simulink model "neha_project"  (Simulink 7.3)
settings: Solver=ode23tb  StartTime=0.0  StopTime=5  RelTol=1000e-2
undefined symbols (not defined in the file): DiscIntNeverNeededParam
libraries: powerlib x16
settings Model: Creator=jassi  LastModifiedBy=ankit
settings SolverCC: ShapePreserveControl=EnableAll  ZeroCrossControl=DisableAll

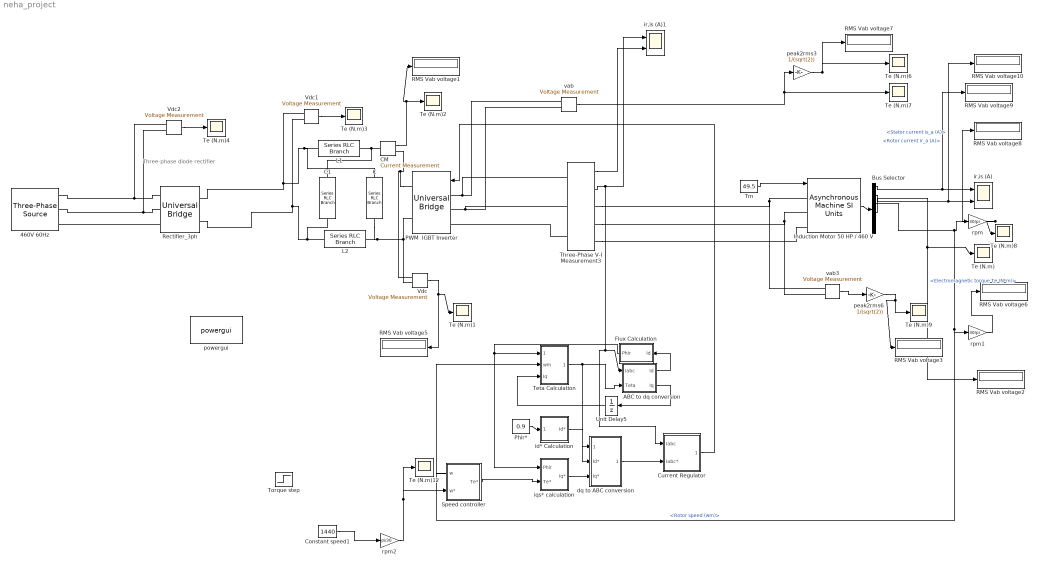
== system neha_project ==
  note: Three-phase
      | diode rectifier
  460V 60Hz : powerlib/Electrical Sources/Three-Phase Source  DialogController=POWERSYS.PowerSysDialog  SystemSampleTime=-1  Voltage=460  PhaseAngle=0  Frequency=50  InternalConnection=Yg  SpecifyImpedance=off  Resistance=0.1  Inductance=1.2e-3  ShortCircuitLevel=100e6  BaseVoltage=25e3  XRratio=7
  ABC to dq conversion : Subsystem
  Bus Selector : BusSelector  OutputSignals=Rotor measurements.Rotor current ir_a (A),Stator measurements.Stator current is_a (A),Mechanical.Rotor speed (wm),Mechanical.Electromagnetic torque Te (N*m),Stator measurements.Stator flux phis_q (V s),Stator measurements.Stator flux phis_d (V s)
  "C " : powerlib/Elements/Series RLC Branch  DialogController=POWERSYS.PowerSysDialog  PhysicalDomain=powersysdomain  SubClassName=unknown  LeftPortType=p1  RightPortType=p1  LConnTagsString=__new0  RConnTagsString=__new0  BranchType=C  Resistance=1  Inductance=1e-3  SetiL0=off  InitialCurrent=0  Capacitance=0.05  Setx0=off  InitialVoltage=0  Measurements=None
  "C1 " : powerlib/Elements/Series RLC Branch  DialogController=POWERSYS.PowerSysDialog  PhysicalDomain=powersysdomain  SubClassName=unknown  LeftPortType=p1  RightPortType=p1  LConnTagsString=__new0  RConnTagsString=__new0  BranchType=C  Resistance=1  Inductance=1e-3  SetiL0=off  InitialCurrent=0  Capacitance=0.05  Setx0=off  InitialVoltage=0  Measurements=None
  CM : powerlib/Measurements/Current Measurement  DialogController=POWERSYS.PowerSysDialog  SystemSampleTime=-1  PhasorSimulation=off  OutputType=Complex  PSBequivalent=0
  Constant speed1 : Constant  Value=1440  OutDataType=sfix(16)  OutScaling=2^0
  Current Regulator : Subsystem  mask(Regulateur de courant a hysteresis){h=20}
      mask prompts: h "Hysteresis band (A)"
  Flux Calculation : Subsystem  mask(Flux Calcultation){}
      mask init:
      | NF=0.44572610323020e-6;
      | DF=[1 -0.99998715486734];
  Induction Motor 50 HP / 460 V : powerlib/Machines/Asynchronous Machine SI Units  DialogController=POWERSYS.PowerSysDialog  SystemSampleTime=-1  PresetModel=No  MechanicalLoad=Torque Tm  ShowDetailedParameters=on  RotorType=Squirrel-cage  ReferenceFrame=Stationary  NominalParameters=[ 7.5e3, 460,50]  Stator=[ 0.6 4.5e-3 ]  Rotor=[ 0.7 4.5e-3 ]  Lm=80e-3  Mechanical=[0.1 0.01 2 ]  PolePairs=2  InitialConditions="[ 1, 0 ,  0 , 0 , 0 , 0 , 0 , 0 ]"  Units=SI  LoadFlowParameters=0  SimulateSaturation=off  Saturation=[0 0;0 0]  TsPowergui=0  TsBlock=-1  IterativeModel=Trapezoidal non iterative
  L1 : powerlib/Elements/Series RLC Branch  DialogController=POWERSYS.PowerSysDialog  PhysicalDomain=powersysdomain  SubClassName=unknown  LeftPortType=p1  RightPortType=p1  LConnTagsString=__new0  RConnTagsString=__new0  BranchType=L  Resistance=1  Inductance=4e-9  SetiL0=off  InitialCurrent=0  Capacitance=1e-6  Setx0=off  InitialVoltage=0  Measurements=None
  L2 : powerlib/Elements/Series RLC Branch  DialogController=POWERSYS.PowerSysDialog  PhysicalDomain=powersysdomain  SubClassName=unknown  LeftPortType=p1  RightPortType=p1  LConnTagsString=__new0  RConnTagsString=__new0  BranchType=L  Resistance=1  Inductance=4e-9  SetiL0=off  InitialCurrent=0  Capacitance=1e-6  Setx0=off  InitialVoltage=0  Measurements=None
  PWM  IGBT Inverter : powerlib/Power Electronics/Universal Bridge  DialogController=POWERSYS.PowerSysDialog  SystemSampleTime=-1  Arms=3  SnubberResistance=1000  SnubberCapacitance=inf  Device=IGBT / Diodes  Ron=1e-3  Lon=0  ForwardVoltages="[  0.0  0.0  ]"  ForwardVoltage=.8  GTOparameters=[ 1e-6 ,1e-6 ]  IGBTparameters=[ 1e-6 , 2.144e-6 ]  Measurements=None  Measurements_2=None  converterType=Rectifier
  Phir* : Constant  Value=0.9  OutDataType=sfix(16)  OutScaling=2^0
  RMS Vab voltage{1..3,5..10} (9 alike) : Display
      settings: Decimation=100
  Rectifier_3ph : powerlib/Power Electronics/Universal Bridge  DialogController=POWERSYS.PowerSysDialog  SystemSampleTime=-1  Arms=3  SnubberResistance=10e3  SnubberCapacitance=20e-9  Device=Diodes  Ron=1e-3  Lon=0  ForwardVoltages="[  0,  0  ]"  ForwardVoltage=1.3  GTOparameters=[ 10e-6, 20e-6 ]  IGBTparameters=[ 1e-6 , 2e-6 ]  Measurements=All voltages and currents  Measurements_2=None  converterType=Rectifier
  Speed controller : Subsystem  mask(PI controller){Kp=4, Ki=200, Tlim=200, Ts=2e-006}
      mask prompts: Kp "Proportional gain (Kp)"; Ki "Integral gain (Ki)"; Tlim "Torque limit (N.m)"; Ts "Sampling time (s)"
      mask help: Proportional-Integral Speed Controller
      mask Display: plot(0,0,100,100,[35,35,65],[70,30,30],[35,65],[45,60])
  Te (N.m){,1..4,6..9,12} (10 alike) : Scope
      Te (N.m) settings: YMin=20  YMax=75  SaveName=ScopeData2  DataFormat=Structure
      Te (N.m)1 settings: YMin=510  YMax=690  SaveName=ScopeData8  DataFormat=Structure
      Te (N.m)12 settings: YMin=120  YMax=120  SaveName=ScopeData16  DataFormat=Structure
      Te (N.m)2 settings: YMin=-40  YMax=60  SaveName=ScopeData9  DataFormat=Structure
      Te (N.m)3 settings: YMin=588  YMax=603  SaveName=ScopeData10  DataFormat=Structure
      Te (N.m)4 settings: YMin=-450  YMax=450  SaveName=ScopeData3  DataFormat=Structure
      Te (N.m)6 settings: YMin=-450  YMax=25  SaveName=ScopeData12  DataFormat=Structure
      Te (N.m)7 settings: YMin=-700  YMax=700  SaveName=ScopeData13  DataFormat=Structure
      Te (N.m)8 settings: TimeRange=1  YMin=550  YMax=1600  DataFormat=Structure
      Te (N.m)9 settings: TimeRange=1  YMin=-400  YMax=400  SaveName=ScopeData14  DataFormat=Structure
  Teta Calculation : Subsystem
  Three-Phase V-I Measurement3 : powerlib/Measurements/Three-Phase V-I Measurement  DialogController=POWERSYS.PowerSysDialog  SystemSampleTime=-1  VoltageMeasurement=phase-to-phase  SetLabelV=off  LabelV=Vabc  Vpu=off  CurrentMeasurement=yes  SetLabelI=off  LabelI=Iabc  Ipu=off  Pbase=100e6  Vbase=500e3  OutputType=Complex  PhasorSimulation=off  PSBequivalent=0
  Tm : Constant  Value=49.5  OutDataType=sfix(16)  OutScaling=2^0
  Torque step : Step  Time=1.8  After=200  SampleTime=0
  Unit Delay5 : UnitDelay  SampleTime=2e-006
  Vdc : powerlib/Measurements/Voltage Measurement  Tag=PoWeRsYsTeMmEaSuReMeNt  DialogController=POWERSYS.PowerSysDialog  SystemSampleTime=-1  PhasorSimulation=off  OutputType=Magnitude  PSBequivalent=0
  Vdc1 : powerlib/Measurements/Voltage Measurement  Tag=PoWeRsYsTeMmEaSuReMeNt  DialogController=POWERSYS.PowerSysDialog  SystemSampleTime=-1  PhasorSimulation=off  OutputType=Magnitude  PSBequivalent=0
  Vdc2 : powerlib/Measurements/Voltage Measurement  Tag=PoWeRsYsTeMmEaSuReMeNt  DialogController=POWERSYS.PowerSysDialog  SystemSampleTime=-1  PhasorSimulation=off  OutputType=Magnitude  PSBequivalent=0
  dq to ABC conversion : Subsystem
  id* Calculation : Subsystem
  iqs* calculation : Subsystem
  ir,is (A) : Scope  NumInputPorts=2
      settings: YMin=-27.5~-55  YMax=17.5~50  DataFormat=Structure
  ir,is (A)1 : Scope  NumInputPorts=2
      settings: YMin=-27.5~-700  YMax=27.5~700  SaveName=ScopeData17  DataFormat=Structure
  peak2rms3 : Gain  Gain=1/(sqrt(2))  ParameterDataType=sfix(16)  ParameterScaling=2^0  OutDataType=sfix(16)  OutScaling=2^0  SaturateOnIntegerOverflow=on  OutDataTypeStr=Inherit: Same as input  ParamDataTypeStr=Inherit: Same as input
  peak2rms6 : Gain  Gain=1/(sqrt(2))  ParameterDataType=sfix(16)  ParameterScaling=2^0  OutDataType=sfix(16)  OutScaling=2^0  SaturateOnIntegerOverflow=on  OutDataTypeStr=Inherit: Same as input  ParamDataTypeStr=Inherit: Same as input
  powergui : powerlib/powergui  Priority=2  SystemSampleTime=-1  SimulationMode=Discrete  SampleTime=2e-006  frequency=60  SPID=off  DisableSnubberDevices=off  DisableRonSwitches=off  DisableVfSwitches=off  SwTol=0  Interpol=off  frequencyindice=50  echomessages=off  HookPort=off  DisplayEquations=off  FunctionMessages=off  EnableUseOfTLC=off  x0status=blocks  RestoreLinks=warning  Frange=[0:2:500]  Ylog=off  Xlog=on  ShowGrid=off  save=off  variable=ZData  ZoomFFT=on  StartTime=0.0  cycles=1  DisplayStyle=off  fundamental=60  FreqAxis=off  MaxFrequency=1000  frequencyindicesteady=1  RmsSteady=1  display=off  Ts=0  methode=off
  rpm : Gain  Gain=30/pi  ParameterDataType=sfix(16)  ParameterScaling=2^0  OutDataType=sfix(16)  OutScaling=2^0  SaturateOnIntegerOverflow=on  OutDataTypeStr=Inherit: Same as input  ParamDataTypeStr=Inherit: Same as input
  rpm1 : Gain  Gain=30/pi  ParameterDataType=sfix(16)  ParameterScaling=2^0  OutDataType=sfix(16)  OutScaling=2^0  SaturateOnIntegerOverflow=on  OutDataTypeStr=Inherit: Same as input  ParamDataTypeStr=Inherit: Same as input
  rpm2 : Gain  Gain=pi/30  ParameterDataType=sfix(16)  ParameterScaling=2^0  OutDataType=sfix(16)  OutScaling=2^0  SaturateOnIntegerOverflow=on  OutDataTypeStr=Inherit: Same as input  ParamDataTypeStr=Inherit: Same as input
  vab : powerlib/Measurements/Voltage Measurement  Tag=PoWeRsYsTeMmEaSuReMeNt  DialogController=POWERSYS.PowerSysDialog  SystemSampleTime=-1  PhasorSimulation=off  OutputType=Magnitude  PSBequivalent=0
  vab3 : powerlib/Measurements/Voltage Measurement  Tag=PoWeRsYsTeMmEaSuReMeNt  DialogController=POWERSYS.PowerSysDialog  SystemSampleTime=-1  PhasorSimulation=off  OutputType=Magnitude  PSBequivalent=0
  wires:
  Bus Selector/4 -> Te (N.m)/1, RMS Vab voltage2/1  "<Electromagnetic torque Te (N*m)>"
  Bus Selector/1 -> RMS Vab voltage9/1, ir,is (A)/1  "<Rotor current ir_a (A)>"
  Induction Motor 50 HP / 460 V/1 -> Bus Selector/1
  Bus Selector/2 -> ir,is (A)/2, RMS Vab voltage10/1  "<Stator current is_a (A)>"
  vab/1 -> peak2rms3/1, Te (N.m)7/1
  Tm/1 -> Induction Motor 50 HP / 460 V/1
  peak2rms3/1 -> Te (N.m)6/1, RMS Vab voltage7/1
  peak2rms6/1 -> RMS Vab voltage3/1, Te (N.m)9/1
  Vdc/1 -> Te (N.m)1/1, RMS Vab voltage5/1
  CM/1 -> Te (N.m)2/1, RMS Vab voltage1/1
  Vdc1/1 -> Te (N.m)3/1
  Three-Phase V-I Measurement3/1 -> ir,is (A)1/2
  Three-Phase V-I Measurement3/2 -> ir,is (A)1/1, Current Regulator/1(Iabc), ABC to dq conversion/1(Iabc)
  vab3/1 -> peak2rms6/1
  Current Regulator/1(Pulses) -> PWM  IGBT Inverter/1
  Bus Selector/3 -> rpm/1, rpm1/1, Teta Calculation/2(wm), Speed controller/1(w)  "<Rotor speed (wm)>"
  rpm/1 -> RMS Vab voltage8/1, Te (N.m)8/1
  rpm1/1 -> RMS Vab voltage6/1
  Teta Calculation/1(Teta) -> dq to ABC conversion/1(Teta), ABC to dq conversion/2(Teta)
  iqs* calculation/1(Iq*) -> dq to ABC conversion/3(Iq*)
  Unit Delay5/1 -> Teta Calculation/3(Iq)
  ABC to dq conversion/2(Iq) -> Unit Delay5/1
  Flux Calculation/1(Phir) -> Teta Calculation/1(Phir), iqs* calculation/1(Phir)
  id* Calculation/1(Id*) -> dq to ABC conversion/2(Id*)
  ABC to dq conversion/1(Id) -> Flux Calculation/1(Id)
  Phir*/1 -> id* Calculation/1(Phir*)
  Speed controller/1(Te*) -> iqs* calculation/2(Te*)
  dq to ABC conversion/1(Iabc*) -> Current Regulator/2(Iabc*)
  rpm2/1 -> Te (N.m)12/1, Speed controller/2(w*)
  Constant speed1/1 -> rpm2/1
  Vdc2/1 -> Te (N.m)4/1
  connections:
  L1/RConn1 -- CM/LConn1 -- "C1 "/LConn1
  Rectifier_3ph/RConn1 -- Vdc1/LConn1 -- L1/LConn1 -- "C "/LConn1
  PWM  IGBT Inverter/RConn2 -- Vdc/LConn2 -- "C "/RConn1 -- L2/RConn1
  Rectifier_3ph/RConn2 -- Vdc1/LConn2 -- L2/LConn1 -- "C1 "/RConn1
  PWM  IGBT Inverter/RConn1 -- Vdc/LConn1 -- CM/RConn1
  Three-Phase V-I Measurement3/RConn2 -- Induction Motor 50 HP / 460 V/LConn2 -- vab3/LConn2
  Three-Phase V-I Measurement3/RConn3 -- Induction Motor 50 HP / 460 V/LConn3
  Three-Phase V-I Measurement3/LConn1 -- PWM  IGBT Inverter/LConn1 -- vab/LConn1
  Three-Phase V-I Measurement3/LConn2 -- vab/LConn2 -- PWM  IGBT Inverter/LConn2
  Three-Phase V-I Measurement3/LConn3 -- PWM  IGBT Inverter/LConn3
  Three-Phase V-I Measurement3/RConn1 -- Induction Motor 50 HP / 460 V/LConn1 -- vab3/LConn1
  460V 60Hz/RConn1 -- Rectifier_3ph/LConn1 -- Vdc2/LConn1
  Rectifier_3ph/LConn3 -- 460V 60Hz/RConn3
  460V 60Hz/RConn2 -- Rectifier_3ph/LConn2 -- Vdc2/LConn2

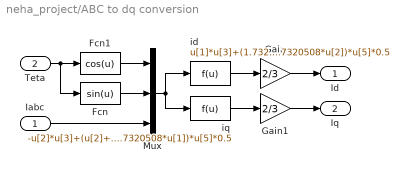
== system neha_project/ABC to dq conversion ==
  Iabc : Inport  OutDataType=sfix(16)  OutScaling=2^0
  Teta : Inport  Port=2  OutDataType=sfix(16)  OutScaling=2^0
  Fcn : Fcn  Expr=sin(u)
  Fcn1 : Fcn  Expr=cos(u)
  Gain : Gain  Gain=2/3  ParameterDataType=sfix(16)  ParameterScaling=2^0  OutDataType=sfix(16)  OutScaling=2^0  SaturateOnIntegerOverflow=on  OutDataTypeStr=Inherit: Same as input  ParamDataTypeStr=Inherit: Same as input
  Gain1 : Gain  Gain=2/3  ParameterDataType=sfix(16)  ParameterScaling=2^0  OutDataType=sfix(16)  OutScaling=2^0  SaturateOnIntegerOverflow=on  OutDataTypeStr=Inherit: Same as input  ParamDataTypeStr=Inherit: Same as input
  Mux : Mux  Inputs=[1 1 3]
  id : Fcn  Expr=u[1]*u[3]+(1.7320508*u[2]-u[1])*u[4]*0.5+(-u[1]-1.7320508*u[2])*u[5]*0.5
  iq : Fcn  Expr=-u[2]*u[3]+(u[2]+1.7320508*u[1])*u[4]*0.5+(u[2]-1.7320508*u[1])*u[5]*0.5
  Id : Outport  OutDataType=sfix(16)  OutScaling=2^0  InitialOutput=0
  Iq : Outport  Port=2  OutDataType=sfix(16)  OutScaling=2^0  InitialOutput=0
  wires:
  Fcn/1 -> Mux/2
  Fcn1/1 -> Mux/1
  Teta/1 -> Fcn1/1, Fcn/1
  Mux/1 -> iq/1, id/1
  Iabc/1 -> Mux/3
  iq/1 -> Gain1/1
  id/1 -> Gain/1
  Gain/1 -> Id/1
  Gain1/1 -> Iq/1

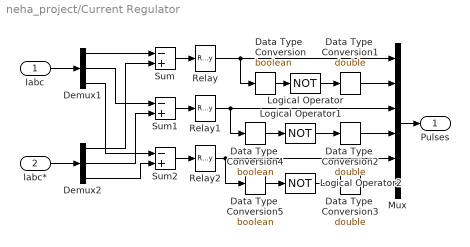
== system neha_project/Current Regulator ==
  Iabc : Inport  OutDataType=sfix(16)  OutScaling=2^0
  Iabc* : Inport  Port=2  OutDataType=sfix(16)  OutScaling=2^0
  Data Type  Conversion : DataTypeConversion  OutDataTypeMode=boolean  OutDataType=sfix(16)  OutScaling=2^0  OutDataTypeStr=boolean  SaturateOnIntegerOverflow=on  RndMeth=Zero
  Data Type  Conversion1 : DataTypeConversion  OutDataTypeMode=double  OutDataType=sfix(16)  OutScaling=2^0  OutDataTypeStr=double  SaturateOnIntegerOverflow=on  RndMeth=Zero
  Data Type  Conversion2 : DataTypeConversion  OutDataTypeMode=double  OutDataType=sfix(16)  OutScaling=2^0  OutDataTypeStr=double  SaturateOnIntegerOverflow=on  RndMeth=Zero
  Data Type  Conversion3 : DataTypeConversion  OutDataTypeMode=double  OutDataType=sfix(16)  OutScaling=2^0  OutDataTypeStr=double  SaturateOnIntegerOverflow=on  RndMeth=Zero
  Data Type  Conversion4 : DataTypeConversion  OutDataTypeMode=boolean  OutDataType=sfix(16)  OutScaling=2^0  OutDataTypeStr=boolean  SaturateOnIntegerOverflow=on  RndMeth=Zero
  Data Type  Conversion5 : DataTypeConversion  OutDataTypeMode=boolean  OutDataType=sfix(16)  OutScaling=2^0  OutDataTypeStr=boolean  SaturateOnIntegerOverflow=on  RndMeth=Zero
  Demux1 : Demux  Outputs=3
  Demux2 : Demux  Outputs=3
  Logical Operator : Logic  Operator=NOT
  Logical Operator1 : Logic  Operator=NOT
  Logical Operator2 : Logic  Operator=NOT
  Mux : Mux  Inputs=6
  Relay : Relay  OnSwitchValue=h/2  OffSwitchValue=-h/2  OutDataType=sfix(16)  OutScaling=2^0
  Relay1 : Relay  OnSwitchValue=h/2  OffSwitchValue=-h/2  OutDataType=sfix(16)  OutScaling=2^0
  Relay2 : Relay  OnSwitchValue=h/2  OffSwitchValue=-h/2  OutDataType=sfix(16)  OutScaling=2^0
  Sum : Sum  Inputs=-+  OutDataType=sfix(16)  OutScaling=2^0  SaturateOnIntegerOverflow=on  InputSameDT=on  OutDataTypeStr=Inherit: Same as first input
  Sum1 : Sum  Inputs=-+  OutDataType=sfix(16)  OutScaling=2^0  SaturateOnIntegerOverflow=on  InputSameDT=on  OutDataTypeStr=Inherit: Same as first input
  Sum2 : Sum  Inputs=-+  OutDataType=sfix(16)  OutScaling=2^0  SaturateOnIntegerOverflow=on  InputSameDT=on  OutDataTypeStr=Inherit: Same as first input
  Pulses : Outport  OutDataType=sfix(16)  OutScaling=2^0  InitialOutput=0
  wires:
  Sum/1 -> Relay/1
  Sum1/1 -> Relay1/1
  Demux1/1 -> Sum/1
  Demux1/2 -> Sum1/1
  Mux/1 -> Pulses/1
  Iabc/1 -> Demux1/1
  Sum2/1 -> Relay2/1
  Demux1/3 -> Sum2/1
  Demux2/3 -> Sum2/2
  Demux2/2 -> Sum1/2
  Demux2/1 -> Sum/2
  Iabc*/1 -> Demux2/1
  Relay/1 -> Mux/1, Data Type  Conversion/1
  Relay1/1 -> Mux/3, Data Type  Conversion4/1
  Relay2/1 -> Mux/5, Data Type  Conversion5/1
  Data Type  Conversion/1 -> Logical Operator/1
  Logical Operator/1 -> Data Type  Conversion1/1
  Data Type  Conversion1/1 -> Mux/2
  Logical Operator1/1 -> Data Type  Conversion2/1
  Data Type  Conversion2/1 -> Mux/4
  Logical Operator2/1 -> Data Type  Conversion3/1
  Data Type  Conversion3/1 -> Mux/6
  Data Type  Conversion4/1 -> Logical Operator1/1
  Data Type  Conversion5/1 -> Logical Operator2/1

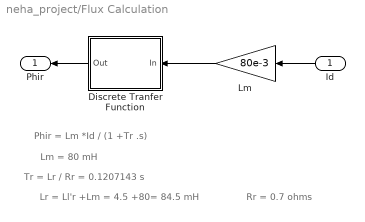
== system neha_project/Flux Calculation ==
  note: Phir = Lm *Id / (1 +Tr .s)
  note: Lm = 80 mH
  note: Lr = Ll'r +Lm = 4.5 +80= 84.5 mH
  note: Tr = Lr / Rr = 0.1207143 s
  note: Rr = 0.7 ohms
  Id : Inport  OutDataType=sfix(16)  OutScaling=2^0
  Discrete Tranfer Function : Subsystem  mask(First Order Low Pass Filter (Discrete)){T=0.1207143, Ts=2e-006}
      mask prompts: T "Time constant T (s) :"; Ts "Time step (s)"
      mask help: H(s)=1/(1+T.s)
      mask init:
      | X=[0 1 2 3 4];
      |  Y=[-2 -2 -3 -4 -4];
      |  str=sprintf('\nH=1/(1+T.s)\n T= %g s\n\n\n',T);
      | num=1;
      | den=[T 1];
      | 
      | % discrete transfer function
      | % descending powers of z
      | numd= Ts/T;
      | dend=[ 1  (Ts-T)/T];
      mask Display:
      | plot(X,Y);
      | disp(str);
  Lm : Gain  Gain=80e-3  ParameterDataType=sfix(16)  ParameterScaling=2^0  OutDataType=sfix(16)  OutScaling=2^0  SaturateOnIntegerOverflow=on  OutDataTypeStr=Inherit: Same as input  ParamDataTypeStr=Inherit: Same as input
  Phir : Outport  OutDataType=sfix(16)  OutScaling=2^0
  wires:
  Discrete Tranfer Function/1(Out) -> Phir/1
  Id/1 -> Lm/1
  Lm/1 -> Discrete Tranfer Function/1(In)

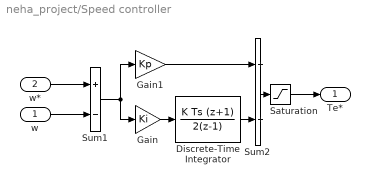
== system neha_project/Speed controller ==
  w : Inport  OutDataType=sfix(16)  OutScaling=2^0
  w* : Inport  Port=2  OutDataType=sfix(16)  OutScaling=2^0
  Discrete-Time Integrator : DiscreteIntegrator  IntegratorMethod=Integration: Trapezoidal  SampleTime=Ts  OutDataType=sfix(16)  OutScaling=2^0  LimitOutput=on  UpperSaturationLimit=Tlim  LowerSaturationLimit=-Tlim  ICPrevOutput=DiscIntNeverNeededParam  ICPrevScaledInput=DiscIntNeverNeededParam
  Gain : Gain  Gain=Ki  ParameterDataType=sfix(16)  ParameterScaling=2^0  OutDataType=sfix(16)  OutScaling=2^0  SaturateOnIntegerOverflow=on  OutDataTypeStr=Inherit: Same as input  ParamDataTypeStr=Inherit: Same as input
  Gain1 : Gain  Gain=Kp  ParameterDataType=sfix(16)  ParameterScaling=2^0  OutDataType=sfix(16)  OutScaling=2^0  SaturateOnIntegerOverflow=on  OutDataTypeStr=Inherit: Same as input  ParamDataTypeStr=Inherit: Same as input
  Saturation : Saturate  UpperLimit=Tlim  LowerLimit=-Tlim
  Sum1 : Sum  Inputs=+-  OutDataType=sfix(16)  OutScaling=2^0  SaturateOnIntegerOverflow=on  InputSameDT=on  OutDataTypeStr=Inherit: Same as first input
  Sum2 : Sum  OutDataType=sfix(16)  OutScaling=2^0  SaturateOnIntegerOverflow=on  InputSameDT=on  OutDataTypeStr=Inherit: Same as first input
  Te* : Outport  OutDataType=sfix(16)  OutScaling=2^0  InitialOutput=0
  wires:
  Gain1/1 -> Sum2/1
  Gain/1 -> Discrete-Time Integrator/1
  Sum1/1 -> Gain/1, Gain1/1
  Discrete-Time Integrator/1 -> Sum2/2
  Sum2/1 -> Saturation/1
  Saturation/1 -> Te*/1
  w/1 -> Sum1/2
  w*/1 -> Sum1/1

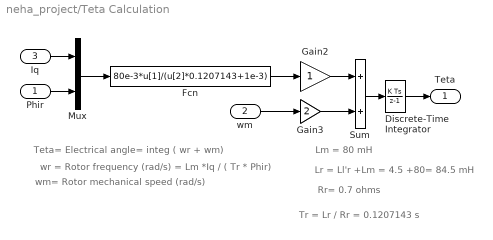
== system neha_project/Teta Calculation ==
  note: Teta= Electrical angle= integ ( wr + wm)
  note: wr = Rotor frequency (rad/s) = Lm *Iq / ( Tr * Phir)
  note: Lm = 80 mH
  note: Rr= 0.7 ohms
  note: Lr = Ll'r +Lm = 4.5 +80= 84.5 mH
  note: wm= Rotor mechanical speed (rad/s)
  note: Tr = Lr / Rr = 0.1207143 s
  Phir : Inport  OutDataType=sfix(16)  OutScaling=2^0
  wm : Inport  Port=2  OutDataType=sfix(16)  OutScaling=2^0
  Iq : Inport  Port=3  OutDataType=sfix(16)  OutScaling=2^0
  Discrete-Time Integrator : DiscreteIntegrator  SampleTime=2e-6  OutDataType=sfix(16)  OutScaling=2^0  ICPrevOutput=DiscIntNeverNeededParam  ICPrevScaledInput=DiscIntNeverNeededParam
  Fcn : Fcn  Expr=80e-3*u[1]/(u[2]*0.1207143+1e-3)
  Gain2 : Gain  ParameterDataType=sfix(16)  ParameterScaling=2^0  OutDataType=sfix(16)  OutScaling=2^0  SaturateOnIntegerOverflow=on  OutDataTypeStr=Inherit: Same as input  ParamDataTypeStr=Inherit: Same as input
  Gain3 : Gain  Gain=2  ParameterDataType=sfix(16)  ParameterScaling=2^0  OutDataType=sfix(16)  OutScaling=2^0  SaturateOnIntegerOverflow=on  OutDataTypeStr=Inherit: Same as input  ParamDataTypeStr=Inherit: Same as input
  Mux : Mux  Inputs=2
  Sum : Sum  OutDataType=sfix(16)  OutScaling=2^0  SaturateOnIntegerOverflow=on  InputSameDT=on  OutDataTypeStr=Inherit: Same as first input
  Teta : Outport  OutDataType=sfix(16)  OutScaling=2^0  InitialOutput=0
  wires:
  Discrete-Time Integrator/1 -> Teta/1
  Sum/1 -> Discrete-Time Integrator/1
  Gain3/1 -> Sum/2
  Gain2/1 -> Sum/1
  wm/1 -> Gain3/1
  Fcn/1 -> Gain2/1
  Phir/1 -> Mux/2
  Iq/1 -> Mux/1
  Mux/1 -> Fcn/1

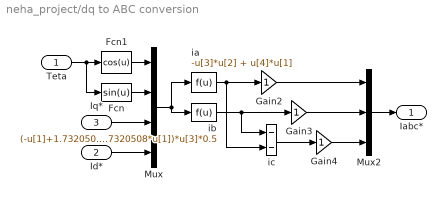
== system neha_project/dq to ABC conversion ==
  Teta : Inport  OutDataType=sfix(16)  OutScaling=2^0
  Id* : Inport  Port=2  OutDataType=sfix(16)  OutScaling=2^0
  Iq* : Inport  Port=3  OutDataType=sfix(16)  OutScaling=2^0
  Fcn : Fcn  Expr=sin(u)
  Fcn1 : Fcn  Expr=cos(u)
  Gain2 : Gain  ParameterDataType=sfix(16)  ParameterScaling=2^0  OutDataType=sfix(16)  OutScaling=2^0  SaturateOnIntegerOverflow=on  OutDataTypeStr=Inherit: Same as input  ParamDataTypeStr=Inherit: Same as input
  Gain3 : Gain  ParameterDataType=sfix(16)  ParameterScaling=2^0  OutDataType=sfix(16)  OutScaling=2^0  SaturateOnIntegerOverflow=on  OutDataTypeStr=Inherit: Same as input  ParamDataTypeStr=Inherit: Same as input
  Gain4 : Gain  ParameterDataType=sfix(16)  ParameterScaling=2^0  OutDataType=sfix(16)  OutScaling=2^0  SaturateOnIntegerOverflow=on  OutDataTypeStr=Inherit: Same as input  ParamDataTypeStr=Inherit: Same as input
  Mux : Mux
  Mux2 : Mux  Inputs=3
  ia : Fcn  Expr=-u[3]*u[2] + u[4]*u[1]
  ib : Fcn  Expr=(-u[1]+1.7320508*u[2])*u[4]*0.5+(u[2]+1.7320508*u[1])*u[3]*0.5
  ic : Sum  Inputs=--  OutDataType=sfix(16)  OutScaling=2^0  SaturateOnIntegerOverflow=on  InputSameDT=on  OutDataTypeStr=Inherit: Same as first input
  Iabc* : Outport  OutDataType=sfix(16)  OutScaling=2^0  InitialOutput=0
  wires:
  Fcn/1 -> Mux/2
  Fcn1/1 -> Mux/1
  Mux2/1 -> Iabc*/1
  Mux/1 -> ib/1, ia/1
  Teta/1 -> Fcn1/1, Fcn/1
  Iq*/1 -> Mux/3
  Id*/1 -> Mux/4
  Gain3/1 -> Mux2/2
  ic/1 -> Gain4/1
  Gain4/1 -> Mux2/3
  Gain2/1 -> Mux2/1
  ia/1 -> Gain2/1, ic/2
  ib/1 -> Gain3/1, ic/1

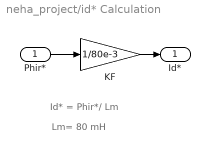
== system neha_project/id* Calculation ==
  note: Id* = Phir*/ Lm
  note: Lm= 80 mH
  Phir* : Inport  OutDataType=sfix(16)  OutScaling=2^0
  KF : Gain  Gain=1/80e-3  ParameterDataType=sfix(16)  ParameterScaling=2^0  OutDataType=sfix(16)  OutScaling=2^0  SaturateOnIntegerOverflow=on  OutDataTypeStr=Inherit: Same as input  ParamDataTypeStr=Inherit: Same as input
  Id* : Outport  OutDataType=sfix(16)  OutScaling=2^0
  wires:
  KF/1 -> Id*/1
  Phir*/1 -> KF/1

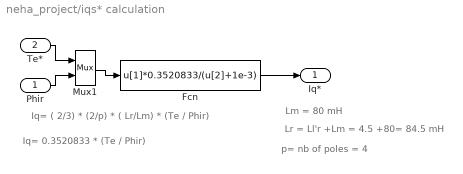
== system neha_project/iqs* calculation ==
  note: Iq= ( 2/3) * (2/p) * ( Lr/Lm) * (Te / Phir)
  note: Lm = 80 mH
  note: Lr = Ll'r +Lm = 4.5 +80= 84.5 mH
  note: p= nb of poles = 4
  note: Iq= 0.3520833 * (Te / Phir)
  Phir : Inport  OutDataType=sfix(16)  OutScaling=2^0
  Te* : Inport  Port=2  OutDataType=sfix(16)  OutScaling=2^0
  Fcn : Fcn  Expr=u[1]*0.3520833/(u[2]+1e-3)
  Mux1 : Mux  Inputs=2
  Iq* : Outport  OutDataType=sfix(16)  OutScaling=2^0  InitialOutput=0
  wires:
  Phir/1 -> Mux1/2
  Fcn/1 -> Iq*/1
  Te*/1 -> Mux1/1
  Mux1/1 -> Fcn/1

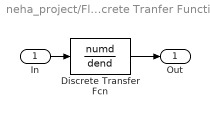
== system neha_project/Flux Calculation/Discrete Tranfer Function ==
  In : Inport  OutDataType=sfix(16)  OutScaling=2^0
  Discrete Transfer Fcn : DiscreteTransferFcn  Numerator=numd  Denominator=dend  SampleTime=Ts
  Out : Outport  OutDataType=sfix(16)  OutScaling=2^0  InitialOutput=0
  wires:
  Discrete Transfer Fcn/1 -> Out/1
  In/1 -> Discrete Transfer Fcn/1
